simulink model "LIFI_SIMULINK"  (R2026a)
settings: Solver=FixedStepDiscrete  StopTime=1  FixedStep=0.001
InitFcn:
  | assignin('base','msgInputBytes', ...
  |     uint8([72 101 108 108 111 32 76 105 70 105 33 zeros(1,21)]));
undefined symbols (not defined in the file or in its folder): msgInputBytes
settings Model: Creator=darshan  LastModifiedBy=darshan

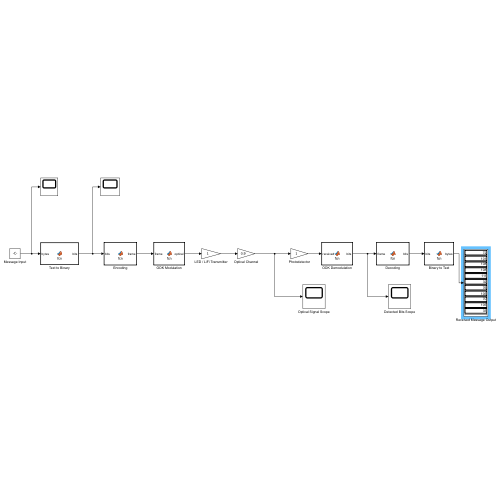
[thumbnail: Simulink's stored preview of the top-level diagram]
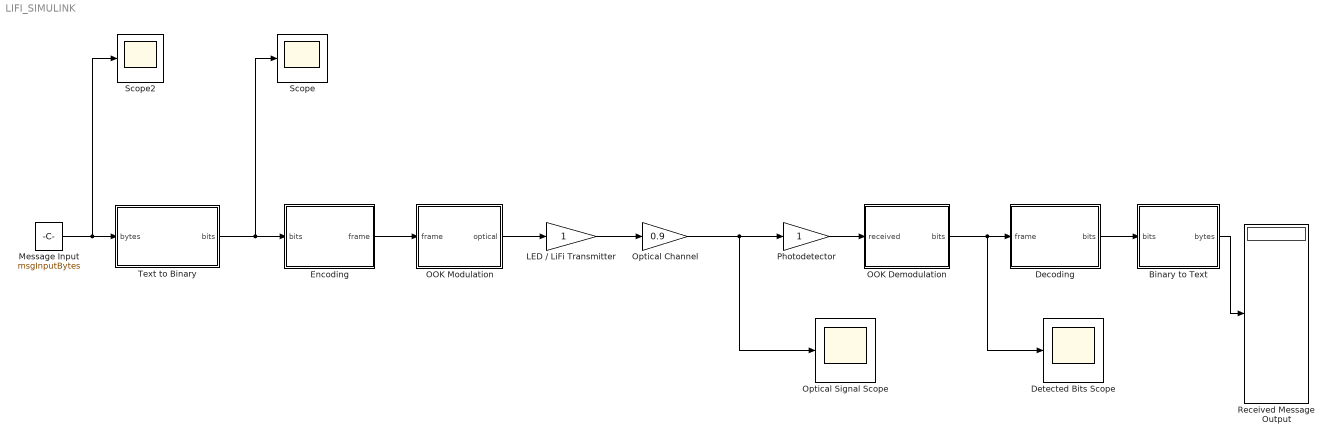
== system LIFI_SIMULINK ==
  Binary to Text : MATLAB Function  TreatAsAtomicUnit=on
  Decoding : MATLAB Function  TreatAsAtomicUnit=on
  Detected Bits Scope : Scope
      settings: ActiveDisplayYMinimum=-1.8792770668655909  ActiveDisplayYMaximum=2.9784788071755544
  Encoding : MATLAB Function  TreatAsAtomicUnit=on
  LED / LiFi Transmitter : Gain
  Message Input : Constant  Value=msgInputBytes  OutDataTypeStr=uint8  SampleTime=-1
  OOK Demodulation : MATLAB Function  TreatAsAtomicUnit=on
  OOK Modulation : MATLAB Function  TreatAsAtomicUnit=on
  Optical Channel : Gain  Gain=0.9
  Optical Signal Scope : Scope
      settings: ActiveDisplayYMinimum=-0.2318806313661006  ActiveDisplayYMaximum=1.3491538671986931
  Photodetector : Gain
  Received Message Output : Display
  Scope : Scope
      settings: ActiveDisplayYMinimum=-2.8731448532293316  ActiveDisplayYMaximum=2.6974767953448904  DataLoggingVariableName=ScopeData2
  Scope2 : Scope
      settings: ActiveDisplayYMinimum=-144.709139492418  ActiveDisplayYMaximum=94.632546993642109  DataLoggingVariableName=ScopeData4
  Text to Binary : MATLAB Function  TreatAsAtomicUnit=on
  wires:
  Message Input/1 -> Scope2/1, Text to Binary/1(bytes)
  Text to Binary/1(bits) -> Encoding/1(bits), Scope/1
  Encoding/1(frame) -> OOK Modulation/1(frame)
  OOK Modulation/1(optical) -> LED / LiFi Transmitter/1
  LED / LiFi Transmitter/1 -> Optical Channel/1
  Optical Channel/1 -> Optical Signal Scope/1, Photodetector/1
  Photodetector/1 -> OOK Demodulation/1(received)
  OOK Demodulation/1(bits) -> Detected Bits Scope/1, Decoding/1(frame)
  Decoding/1(bits) -> Binary to Text/1(bits)
  Binary to Text/1(bytes) -> Received Message Output/1

== matlab function LIFI_SIMULINK/Text to Binary ==
  data: bytes input; bits output
function bits = fcn(bytes)
% TEXT TO BINARY
% Converts exactly 32 bytes into 256 binary bits.
% Most significant bit is transmitted first.

bits = zeros(256,1,'uint8');

for k = 1:32

    b = uint8(bytes(k));

    for j = 1:8

        bits((k-1)*8+j) = uint8(bitget(b,9-j));

    end

end

== matlab function LIFI_SIMULINK/OOK Modulation ==
  data: frame input; optical output
function optical = fcn(frame)
% OOK MODULATION
%
% Binary 1 -> LED ON
% Binary 0 -> LED OFF

optical = double(frame);

== matlab function LIFI_SIMULINK/OOK Demodulation ==
  data: received input; bits output
function bits = fcn(received)
% OOK DEMODULATION
%
% Threshold:
% received >= 0.45 -> binary 1
% received <  0.45 -> binary 0

threshold = 0.45;

bits = uint8(received >= threshold);

== matlab function LIFI_SIMULINK/Decoding ==
  data: frame input; bits output
function bits = fcn(frame)
% DECODING / DEFRAMING
%
% Removes:
% 16-bit synchronization preamble
% 1 parity bit after every 8 data bits
%
% Output = original 256 data bits.

bits = zeros(256,1,'uint8');

inIndex = 17;
outIndex = 1;

for k = 1:32

    % Recover 8 data bits
    for j = 1:8

        bits(outIndex) = frame(inIndex);

        inIndex = inIndex + 1;
        outIndex = outIndex + 1;

    end

    % Skip parity bit
    inIndex = inIndex + 1;

end

== matlab function LIFI_SIMULINK/Binary to Text ==
  data: bits input; bytes output
function bytes = fcn(bits)
% BINARY TO TEXT
%
% Converts 256 binary bits into 32 UTF-8/ASCII byte values.

bytes = zeros(32,1,'uint8');

for k = 1:32

    value = uint8(0);

    for j = 1:8

        value = bitor( ...
            value, ...
            bitshift(uint8(bits((k-1)*8+j)),8-j));

    end

    bytes(k) = value;

end

== matlab function LIFI_SIMULINK/Encoding ==
  data: bits input; frame output
function frame = fcn(bits)
% ENCODING / FRAMING
%
% Adds:
% 1. 16-bit synchronization preamble
% 2. One even-parity bit after every 8 data bits
%
% 32 bytes = 256 data bits
% 32 parity bits
% 16 preamble bits
%
% Total transmitted frame = 304 bits.

frame = zeros(304,1,'uint8');

% ---------------------------------------------------------
% 16-bit synchronization preamble
% 1010101010101010
% ---------------------------------------------------------

for k = 1:16
    frame(k) = uint8(mod(k,2)==1);
end

% ---------------------------------------------------------
% Data + parity
% ---------------------------------------------------------

outIndex = 17;

for k = 1:32

    startIndex = (k-1)*8 + 1;

    dataBits = bits(startIndex:startIndex+7);

    % Copy 8 data bits
    for j = 1:8
        frame(outIndex) = dataBits(j);
        outIndex = outIndex + 1;
    end

    % Even parity bit
    parity = uint8(mod(sum(double(dataBits)),2));

    frame(outIndex) = parity;
    outIndex = outIndex + 1;

end
